simulink model "c130JSBSim"  (R2026a)
settings: Solver=ode4  StopTime=inf  FixedStep=stepSize_s
undefined symbols (not defined in the file): actuatorDelay_s, plantSampleTime_s, referenceLatitude_deg, referenceLongitude_deg, vehicleParams
settings Model: Creator=GTAR  LastModifiedBy=Edison Altamirano
settings DebuggingCC: ModelReferenceIOMismatchMessage=warning
settings ModelReferenceCC: ModelReferenceNumInstancesAllowed=Single

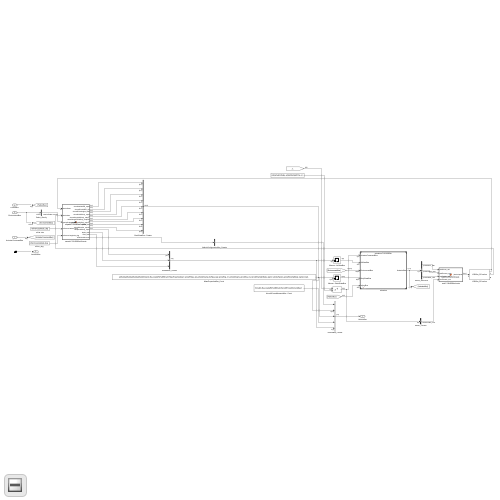
[thumbnail: Simulink's stored preview of the top-level diagram]
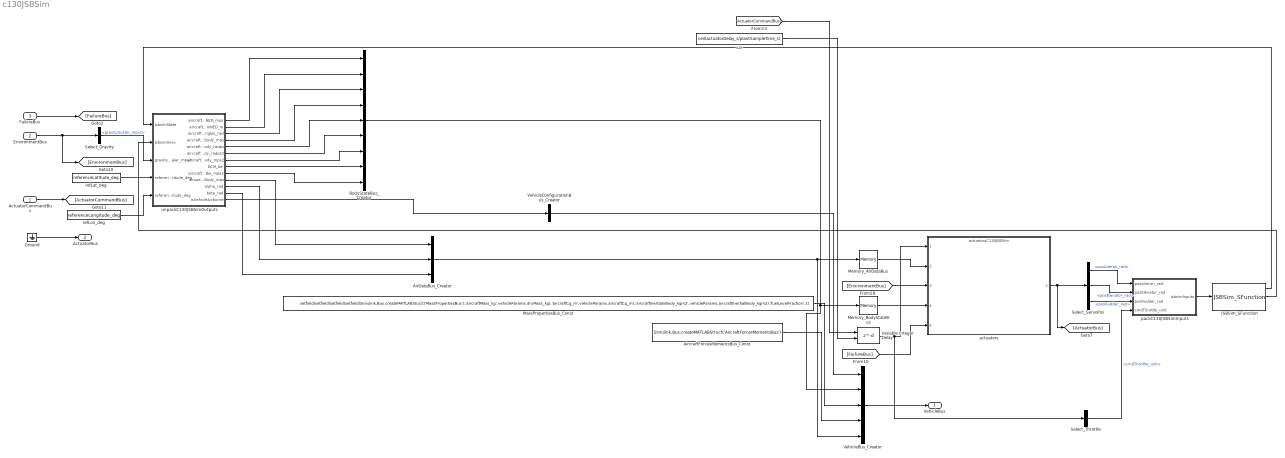
== system c130JSBSim ==
  ActuatorCommandBus : Inport  OutDataTypeStr=Bus: ActuatorCommandBus
  EnvironmentBus : Inport  Port=2  OutDataTypeStr=Bus: EnvironmentBus
  FailureBus : Inport  Port=3  OutDataTypeStr=Bus: FailureBus
  AirDataBus_Creator : BusCreator  Inputs=3  OutDataTypeStr=Bus: AirDataBus
  AircraftForcesMomentsBus_Const : Constant  Value=Simulink.Bus.createMATLABStruct('AircraftForcesMomentsBus')  OutDataTypeStr=Bus: AircraftForcesMomentsBus
  BodyStateBus_Creator : BusCreator  Inputs=9  OutDataTypeStr=Bus: BodyStateBus
  Ground : Ground
  JSBSim_SFunction : S-Function  FunctionName=JSBSim_SFunction  Parameters='C130', stepSize_s, 0, '', 'c130JSBSimInit', 'C:/Users/Edison Altamirano/SITLV2/AnelloSummer/optimAeroPX4SIL/c130JSBSim_io.xml'  SFunctionDeploymentMode=off  EnableBusSupport=off
  MassPropertiesBus_Const : Constant  Value=setfield(setfield(setfield(setfield(Simulink.Bus.createMATLABStruct('MassPropertiesBus'),'aircraftMass_kg',vehicleParams.dryMass_kg),'aircraftCg_m',vehicleParams.aircraftCg_m),'aircraftInertiaInBody_kgm2',vehicleParams.aircraftInertialBody_kgm2),'fuelLevelFraction',1)  OutDataTypeStr=Bus: MassPropertiesBus
  Memory_AirDataBus : Memory
  Memory_BodyStateBus : Memory
  Select_Gravity : BusSelector  OutputSignals=EarthEnvironment.gravityScalar_mps2
  Select_ServoPos : BusSelector  OutputSignals=ServosBus.ServosFixedwingPlaneBus.posAileron_rad,ServosBus.ServosFixedwingPlaneBus.posElevator_rad,ServosBus.ServosFixedwingPlaneBus.posRudder_rad
  Select_Throttle : BusSelector  OutputSignals=EngineCommandBus.cmdThrottle_unit
  Variable Integer Delay : Delay  DelayLengthSource=Input port
      settings: InputPortMap=u0,p1
  VehicleBus_Creator : BusCreator  Inputs=5  OutDataTypeStr=Bus: VehicleBus
  VehicleConfigurationBus_Creator : BusCreator  Inputs=1  OutDataTypeStr=Bus: VehicleConfigurationBus
  actuators : ModelReference  ModelNameDialog=actuatorsC130JSBSim.slx  SimulationMode=Normal  ModelReferenceVersion=5.3
  packC130JSBSimInputs : MATLAB Function  TreatAsAtomicUnit=on
  refLat_deg : Constant  Value=referenceLatitude_deg
  refLon_deg : Constant  Value=referenceLongitude_deg
  unpackC130JSBSimOutputs : MATLAB Function  TreatAsAtomicUnit=on
  var : Constant  Value=ceil(actuatorDelay_s/plantSampleTime_s)
  VehicleBus : Outport  OutDataTypeStr=Bus: VehicleBus
  ActuatorBus : Outport  Port=2  OutDataTypeStr=Bus: ActuatorBus
  wires:
  [FailureBus] -> actuators/5
  EnvironmentBus/1 -> [EnvironmentBus], Select_Gravity/1
  Variable Integer Delay/1 -> actuators/1, Select_Throttle/1
  [EnvironmentBus] -> actuators/3
  FailureBus/1 -> [FailureBus]
  Select_Gravity/1 -> unpackC130JSBSimOutputs/3(gravityScalar_mps2)  "<gravityScalar_mps2>"
  MassPropertiesBus_Const/1 -> VehicleBus_Creator/3
  ActuatorCommandBus/1 -> [ActuatorCommandBus]
  Ground/1 -> ActuatorBus/1
  unpackC130JSBSimOutputs/1(aircraftVelInNED_mps) -> BodyStateBus_Creator/1
  refLat_deg/1 -> unpackC130JSBSimOutputs/4(referenceLatitude_deg)
  refLon_deg/1 -> unpackC130JSBSimOutputs/5(referenceLongitude_deg)
  unpackC130JSBSimOutputs/3(aircraftEulerAngles_rad) -> BodyStateBus_Creator/3
  unpackC130JSBSimOutputs/2(aircraftPosInNED_m) -> BodyStateBus_Creator/2
  unpackC130JSBSimOutputs/4(aircraftVelInBody_mps) -> BodyStateBus_Creator/4
  unpackC130JSBSimOutputs/5(aircraftAngVelInBody_radps) -> BodyStateBus_Creator/5
  unpackC130JSBSimOutputs/6(aircraftAngAccelInBody_radps2) -> BodyStateBus_Creator/6
  unpackC130JSBSimOutputs/7(aircraftAccelInBody_mps2) -> BodyStateBus_Creator/7
  VehicleConfigurationBus_Creator/1 -> VehicleBus_Creator/1
  unpackC130JSBSimOutputs/8(DCM_be) -> BodyStateBus_Creator/8
  unpackC130JSBSimOutputs/9(aircraftAccelbe_mps2) -> BodyStateBus_Creator/9
  unpackC130JSBSimOutputs/10(airspeedInBody_mps) -> AirDataBus_Creator/1
  unpackC130JSBSimOutputs/11(alpha_rad) -> AirDataBus_Creator/2
  unpackC130JSBSimOutputs/12(beta_rad) -> AirDataBus_Creator/3
  unpackC130JSBSimOutputs/13(isVehicleAirborne) -> VehicleConfigurationBus_Creator/1
  Memory_BodyStateBus/1 -> actuators/4
  [ActuatorCommandBus] -> Variable Integer Delay/1
  packC130JSBSimInputs/1(jsbsimInputs) -> JSBSim_SFunction/1
  var/1 -> Variable Integer Delay/2
  JSBSim_SFunction/2 -> unpackC130JSBSimOutputs/2(jsbsimAero)
  BodyStateBus_Creator/1 -> Memory_BodyStateBus/1, VehicleBus_Creator/2
  AirDataBus_Creator/1 -> Memory_AirDataBus/1, VehicleBus_Creator/5
  AircraftForcesMomentsBus_Const/1 -> VehicleBus_Creator/4
  Memory_AirDataBus/1 -> actuators/2
  Select_ServoPos/2 -> packC130JSBSimInputs/2(posElevator_rad)  "<posElevator_rad>"
  VehicleBus_Creator/1 -> VehicleBus/1
  actuators/1 -> [ActuatorBus], Select_ServoPos/1
  Select_ServoPos/1 -> packC130JSBSimInputs/1(posAileron_rad)  "<posAileron_rad>"
  Select_ServoPos/3 -> packC130JSBSimInputs/3(posRudder_rad)  "<posRudder_rad>"
  JSBSim_SFunction/1 -> unpackC130JSBSimOutputs/1(jsbsimState)
  Select_Throttle/1 -> packC130JSBSimInputs/4(cmdThrottle_unit)  "<cmdThrottle_unit>"

== matlab function c130JSBSim/unpackC130JSBSimOutputs ==
  data: jsbsimState input; aircraftVelInNED_mps output; jsbsimAero input; gravityScalar_mps2 input; referenceLatitude_deg input; referenceLongitude_deg input; aircraftPosInNED_m output; aircraftEulerAngles_rad output; aircraftVelInBody_mps output; aircraftAngVelInBody_radps output; aircraftAngAccelInBody_radps2 output; aircraftAccelInBody_mps2 output; DCM_be output; aircraftAccelbe_mps2 output; airspeedInBody_mps output; alpha_rad output; beta_rad output; isVehicleAirborne output
function [aircraftVelInNED_mps, aircraftPosInNED_m, aircraftEulerAngles_rad, ...
          aircraftVelInBody_mps, aircraftAngVelInBody_radps, aircraftAngAccelInBody_radps2, ...
          aircraftAccelInBody_mps2, DCM_be, aircraftAccelbe_mps2, ...
          airspeedInBody_mps, alpha_rad, beta_rad, isVehicleAirborne] = ...
          unpackC130JSBSimOutputs(jsbsimState, jsbsimAero, gravityScalar_mps2, ...
          referenceLatitude_deg, referenceLongitude_deg) %#codegen
% Converts JSBSim_SFunction's raw English-unit "State"/"Aero" output vectors (see
% c130JSBSim_io.xml for the exact property order this function assumes) into the SI
% BodyStateBus/AirDataBus fields the rest of this SIL expects. Same conversions as
% c172pJSBSim's own unpackJSBSimOutputs.m (aircraft-independent physics -- see
% PLAN_JSBSIM_SFUNCTION_HYBRID_C172P.md §2 for the original derivation of each one); only the
% function/file name differs per PLAN_JSBSIM_SFUNCTION_F22_C130.md Phase C.
%
% jsbsimState order (19): lat-gc-deg, long-gc-deg, h-sl-ft, phi-rad, theta-rad, psi-rad, u-fps,
%   v-fps, w-fps, p-rad_sec, q-rad_sec, r-rad_sec, udot-ft_sec2, vdot-ft_sec2, wdot-ft_sec2,
%   pdot-rad_sec2, qdot-rad_sec2, rdot-rad_sec2, h-agl-ft
% jsbsimAero order (5): alpha-rad, beta-rad, u-aero-fps, v-aero-fps, w-aero-fps
ft2m = 0.3048;

lat_deg     = jsbsimState(1);
lon_deg     = jsbsimState(2);
h_sl_ft     = jsbsimState(3);
phi_rad     = jsbsimState(4);
theta_rad   = jsbsimState(5);
psi_rad     = jsbsimState(6);
u_fps       = jsbsimState(7);
v_fps       = jsbsimState(8);
w_fps       = jsbsimState(9);
p_radps     = jsbsimState(10);
q_radps     = jsbsimState(11);
r_radps     = jsbsimState(12);
udot_ftps2  = jsbsimState(13);
vdot_ftps2  = jsbsimState(14);
wdot_ftps2  = jsbsimState(15);
pdot_radps2 = jsbsimState(16);
qdot_radps2 = jsbsimState(17);
rdot_radps2 = jsbsimState(18);
h_agl_ft    = jsbsimState(19);

alpha_rad = jsbsimAero(1);
beta_rad  = jsbsimAero(2);
u_aero_fps = jsbsimAero(3);
v_aero_fps = jsbsimAero(4);
w_aero_fps = jsbsimAero(5);

% Nav (NED) -> body DCM, standard 3-2-1 Euler sequence (Aerospace Toolbox, codegen-compatible).
DCM_be = angle2dcm(psi_rad, theta_rad, phi_rad);

% Local flat-Earth tangent-plane position, anchored at this vehicle's own reference lat/lon (same
% point setUpVehicle.m's "c130jsbsim" case and c130JSBSimInit.xml use), with zDown absolute
% (-h_sl_ft*ft2m), matching every other vehicle's aircraftInitialPosInNED_m convention. Hand-coded
% spherical equirectangular approximation instead of Aerospace Toolbox's lla2flat -- lla2flat
% breaks Simulink's MATLAB Function block type inference in this MATLAB release (confirmed by
% isolated reproduction during c172pJSBSim's own Phase C, same bug class documented in
% optimAeroPX4SIL/CLAUDE.md section 3). At the sub-100km scale this SIL operates at, the
% spherical/WGS84 difference is negligible.
earthRadius_m = 6371000;
dLat_rad = (lat_deg - referenceLatitude_deg) * pi/180;
dLon_rad = (lon_deg - referenceLongitude_deg) * pi/180;
xNorth_m = dLat_rad * earthRadius_m;
yEast_m = dLon_rad * earthRadius_m * cos(referenceLatitude_deg * pi/180);
zDown_m = -h_sl_ft * ft2m;
aircraftPosInNED_m = [xNorth_m; yEast_m; zDown_m];

aircraftVelInBody_mps = [u_fps; v_fps; w_fps] * ft2m;
aircraftVelInNED_mps = DCM_be' * aircraftVelInBody_mps;

aircraftAngVelInBody_radps = [p_radps; q_radps; r_radps];
aircraftAngAccelInBody_radps2 = [pdot_radps2; qdot_radps2; rdot_radps2];

% JSBSim's accelerations/{u,v,w}dot-ft_sec2 are TOTAL body-axis acceleration at the CG (includes
% gravity's contribution via the equations of motion) -- i.e. the same "raw inertial acceleration"
% quantity every other vehicle's plant supplies for this field. `aircraftAccelbe_mps2` must stay
% the RAW acceleration here, NOT specific force: both ins.slx's "Three-axis Inertial Measurement
% Unit" block (aerolibnav) and ANELLO_X3_IMU_Vehicle_fcn_SIL.m already subtract gravity themselves
% (their own g_body/Gb input) to turn raw acceleration into specific force. Subtracting gravity a
% second time here would double-count it.
%
% CENTRIPETAL/CORIOLIS CORRECTION (2026-08-01, c130run7/8 post-mortem,
% PLAN_JSBSIM_SFUNCTION_F22_C130.md section 13.9): udot/vdot/wdot as JSBSim computes them
% (FGPropagate: vUVWdot = vForces/mass - vPQR x vUVW) are the component-wise derivative of the
% body velocity vector AS SEEN IN THE ROTATING BODY FRAME (dV/dt|_body) -- NOT the true inertial
% acceleration expressed in body axes. By the rotating-frame transport theorem (standard flight
% dynamics, e.g. Stevens & Lewis "Aircraft Control and Simulation"):
%   a_inertial_body = dV/dt|_body + omega x V
% Previously the omega x V term was omitted entirely, so the "raw acceleration" fed to every
% downstream accelerometer/IMU model was silently missing this centripetal/Coriolis coupling
% term -- exactly zero during straight, non-rotating flight (which is why this was never caught
% before), but growing with p/q/r during any coordinated turn, i.e. precisely when this SIL's own
% C130 EKF2 divergence was observed. Not yet confirmed as THE root cause (needs re-test), but this
% is a genuine, first-principles-derived correctness bug independent of that investigation.
omegaCrossV_ftps2 = [q_radps*w_fps - r_radps*v_fps; ...
                     r_radps*u_fps - p_radps*w_fps; ...
                     p_radps*v_fps - q_radps*u_fps];
aircraftAccelInBody_mps2 = ([udot_ftps2; vdot_ftps2; wdot_ftps2] + omegaCrossV_ftps2) * ft2m;
aircraftAccelbe_mps2 = aircraftAccelInBody_mps2;

aircraftEulerAngles_rad = [phi_rad; theta_rad; psi_rad];

% Airmass-relative body-axis velocity (wind-inclusive) for AirDataBus -- NOT the inertial u/v/w.
airspeedInBody_mps = [u_aero_fps; v_aero_fps; w_aero_fps] * ft2m;

isVehicleAirborne = (h_agl_ft * ft2m) > 0.1;
end

== matlab function c130JSBSim/packC130JSBSimInputs ==
  data: posAileron_rad input; jsbsimInputs output; posElevator_rad input; posRudder_rad input; cmdThrottle_unit input
function jsbsimInputs = packC130JSBSimInputs(posAileron_rad, posElevator_rad, posRudder_rad, cmdThrottle_unit)
%#codegen
% Re-normalizes actuatorsC130JSBSim.slx's achieved (rate-limited) surface positions back to
% JSBSim's fcs/*-cmd-norm convention, using the same real deflection limits as
% setUpActuators.m's "c130jsbsim" case (sourced from C130.xml <flight_control> aerosurface_scale
% ranges: elevator -0.35/+0.3 rad, aileron/rudder +-0.35 rad -- symmetric +-0.35 rad/20.05 deg used
% here for all three, same "store/use the larger magnitude" convention as setUpActuators.m).
% Throttle is broadcast to all 4 T56 engine indices -- PX4's MAV_TYPE 1 airframe has only one
% throttle channel, no independent per-engine control in this pass (see
% PLAN_JSBSIM_SFUNCTION_F22_C130.md Phase B). Output order matches c130JSBSim_io.xml <input> order
% exactly: aileron, elevator, rudder, throttle[0], throttle[1], throttle[2], throttle[3],
% gear-cmd-norm, left brake, right brake -- do not reorder without updating that file.
% gear-cmd-norm is a hardcoded 1.0
% (gear permanently down, never retracts) -- see c130JSBSim_io.xml's header comment for why this
% is required (unlike c172p's fixed gear, C130's gear is retractable and defaults to 0/up if left
% undriven, which would remove ground-contact support entirely at simulation start).
maxAilDefl_rad = 20.05 * pi/180;
maxElevatorDefl_rad = 20.05 * pi/180;
maxRudderDefl_rad = 20.05 * pi/180;

aileronCmd_norm = max(min(posAileron_rad / maxAilDefl_rad, 1), -1);
elevatorCmd_norm = max(min(posElevator_rad / maxElevatorDefl_rad, 1), -1);
rudderCmd_norm = max(min(posRudder_rad / maxRudderDefl_rad, 1), -1);
throttleCmd_norm = max(min(cmdThrottle_unit, 1), 0);
gearCmd_norm = 1;
% Running T56 engines produce enough idle thrust to move the aircraft while
% PX4/MAVSDK are still connecting. Hold both main-wheel brakes at idle and
% release them as soon as PX4 commands meaningful takeoff power. Reapplying
% this rule after touchdown also lets PX4 confirm landed/disarmed.
brakeCmd_norm = double(throttleCmd_norm < 0.05);

jsbsimInputs = [aileronCmd_norm; elevatorCmd_norm; rudderCmd_norm; ...
                throttleCmd_norm; throttleCmd_norm; throttleCmd_norm; throttleCmd_norm; ...
                gearCmd_norm; brakeCmd_norm; brakeCmd_norm];
end
